simulink library "ammclib_bam_s32k14x"  (Simulink 9.0)
settings: Solver=ode45  StartTime=0.0  StopTime=10.0  RelTol=1e-3
undefined symbols (not defined in the file): f16A1, f16A2, f16B0, f16B1, f16B2, f16C1, f16CC1, f16CC1sc, f16CC1sc_D, f16CC1sc_Q, f16CC1scD, f16CC1scQ, f16CC2, f16CC2sc, f16CC2sc_D, f16CC2sc_Q, f16CC2scD, f16CC2scQ, f16DerivGain, f16EGain, f16FiltCoef, f16HystOff, f16HystOn, f16IGain, f16IntegGain, f16IntegGainFW, f16IntegGainQ, f16Kd, f16Kq, f16Limit, f16LowerLim, f16LowerLimit_D, f16LowerLimit_Q, f16ModIndex, f16OutValOff, f16OutValOn, f16PropGain, f16PropGainFW, f16PropGainQ, f16RampDown, f16RampUp, f16UGain, f16UpperLim, f16UpperLimit, f16UpperLimit_D, f16UpperLimit_Q, f16WIGain, f32A1, f32A2, f32B0, f32B1, f32B2, f32C1, f32CC1, f32CC1sc, f32CC1sc_D, f32CC1sc_Q, f32CC1scD, f32CC1scQ, f32CC2 ... (+122)
(part 11 of 11)

== system ammclib_bam_s32k14x/MLIB/bam_f32f16f16/MLIB_Msu_F32F16F16/copyright2 ==

== system ammclib_bam_s32k14x/MLIB/bam_f32f16f16/MLIB_Msu_F32F16F16/logo ==

== system ammclib_bam_s32k14x/MLIB/bam_f32f16f16/MLIB_MulSat_F32F16F16/copyright ==

== system ammclib_bam_s32k14x/MLIB/bam_f32f16f16/MLIB_MulSat_F32F16F16/copyright2 ==

== system ammclib_bam_s32k14x/MLIB/bam_f32f16f16/MLIB_MulSat_F32F16F16/logo ==

== system ammclib_bam_s32k14x/MLIB/bam_f32f16f16/MLIB_Mul_F32F16F16/copyright ==

== system ammclib_bam_s32k14x/MLIB/bam_f32f16f16/MLIB_Mul_F32F16F16/copyright2 ==

== system ammclib_bam_s32k14x/MLIB/bam_f32f16f16/MLIB_Mul_F32F16F16/logo ==

== system ammclib_bam_s32k14x/MLIB/bam_f32f16f16/MLIB_VMac_F32F16F16/copyright ==

== system ammclib_bam_s32k14x/MLIB/bam_f32f16f16/MLIB_VMac_F32F16F16/copyright2 ==

== system ammclib_bam_s32k14x/MLIB/bam_f32f16f16/MLIB_VMac_F32F16F16/logo ==

== system ammclib_bam_s32k14x/MLIB/bam_flt/MLIB_Abs_FLT/copyright ==

== system ammclib_bam_s32k14x/MLIB/bam_flt/MLIB_Abs_FLT/copyright2 ==

== system ammclib_bam_s32k14x/MLIB/bam_flt/MLIB_Abs_FLT/logo ==

== system ammclib_bam_s32k14x/MLIB/bam_flt/MLIB_Add_FLT/copyright ==

== system ammclib_bam_s32k14x/MLIB/bam_flt/MLIB_Add_FLT/copyright2 ==

== system ammclib_bam_s32k14x/MLIB/bam_flt/MLIB_Add_FLT/logo ==

== system ammclib_bam_s32k14x/MLIB/bam_flt/MLIB_ConvertPU_FLTF16/copyright ==

== system ammclib_bam_s32k14x/MLIB/bam_flt/MLIB_ConvertPU_FLTF16/copyright2 ==

== system ammclib_bam_s32k14x/MLIB/bam_flt/MLIB_ConvertPU_FLTF16/logo ==

== system ammclib_bam_s32k14x/MLIB/bam_flt/MLIB_ConvertPU_FLTF32/copyright ==

== system ammclib_bam_s32k14x/MLIB/bam_flt/MLIB_ConvertPU_FLTF32/copyright2 ==

== system ammclib_bam_s32k14x/MLIB/bam_flt/MLIB_ConvertPU_FLTF32/logo ==

== system ammclib_bam_s32k14x/MLIB/bam_flt/MLIB_Convert_FLTF16/copyright ==

== system ammclib_bam_s32k14x/MLIB/bam_flt/MLIB_Convert_FLTF16/copyright2 ==

== system ammclib_bam_s32k14x/MLIB/bam_flt/MLIB_Convert_FLTF16/logo ==

== system ammclib_bam_s32k14x/MLIB/bam_flt/MLIB_Convert_FLTF32/copyright ==

== system ammclib_bam_s32k14x/MLIB/bam_flt/MLIB_Convert_FLTF32/copyright2 ==

== system ammclib_bam_s32k14x/MLIB/bam_flt/MLIB_Convert_FLTF32/logo ==

== system ammclib_bam_s32k14x/MLIB/bam_flt/MLIB_Div_FLT/copyright ==

== system ammclib_bam_s32k14x/MLIB/bam_flt/MLIB_Div_FLT/copyright2 ==

== system ammclib_bam_s32k14x/MLIB/bam_flt/MLIB_Div_FLT/logo ==

== system ammclib_bam_s32k14x/MLIB/bam_flt/MLIB_Mac_FLT/copyright ==

== system ammclib_bam_s32k14x/MLIB/bam_flt/MLIB_Mac_FLT/copyright2 ==

== system ammclib_bam_s32k14x/MLIB/bam_flt/MLIB_Mac_FLT/logo ==

== system ammclib_bam_s32k14x/MLIB/bam_flt/MLIB_Mnac_FLT/copyright ==

== system ammclib_bam_s32k14x/MLIB/bam_flt/MLIB_Mnac_FLT/copyright2 ==

== system ammclib_bam_s32k14x/MLIB/bam_flt/MLIB_Mnac_FLT/logo ==

== system ammclib_bam_s32k14x/MLIB/bam_flt/MLIB_Msu_FLT/copyright ==

== system ammclib_bam_s32k14x/MLIB/bam_flt/MLIB_Msu_FLT/copyright2 ==

== system ammclib_bam_s32k14x/MLIB/bam_flt/MLIB_Msu_FLT/logo ==

== system ammclib_bam_s32k14x/MLIB/bam_flt/MLIB_Mul_FLT/copyright ==

== system ammclib_bam_s32k14x/MLIB/bam_flt/MLIB_Mul_FLT/copyright2 ==

== system ammclib_bam_s32k14x/MLIB/bam_flt/MLIB_Mul_FLT/logo ==

== system ammclib_bam_s32k14x/MLIB/bam_flt/MLIB_Neg_FLT/copyright ==

== system ammclib_bam_s32k14x/MLIB/bam_flt/MLIB_Neg_FLT/copyright2 ==

== system ammclib_bam_s32k14x/MLIB/bam_flt/MLIB_Neg_FLT/logo ==

== system ammclib_bam_s32k14x/MLIB/bam_flt/MLIB_Sub_FLT/copyright ==

== system ammclib_bam_s32k14x/MLIB/bam_flt/MLIB_Sub_FLT/copyright2 ==

== system ammclib_bam_s32k14x/MLIB/bam_flt/MLIB_Sub_FLT/logo ==

== system ammclib_bam_s32k14x/MLIB/bam_flt/MLIB_VMac_FLT/copyright ==

== system ammclib_bam_s32k14x/MLIB/bam_flt/MLIB_VMac_FLT/copyright2 ==

== system ammclib_bam_s32k14x/MLIB/bam_flt/MLIB_VMac_FLT/logo ==

== system ammclib_bam_s32k14x/GFLIB/bam_flt/GFLIB_VLog10_FLT/GFLIB_VLog10_FLT/copyright ==

== system ammclib_bam_s32k14x/GFLIB/bam_flt/GFLIB_VLog10_FLT/GFLIB_VLog10_FLT/copyright2 ==

== system ammclib_bam_s32k14x/GFLIB/bam_flt/GFLIB_VLog10_FLT/GFLIB_VLog10_FLT/logo ==
